simulink model "MAXPID_modelisation_multi_physique_MATLAB_2015a_Ivan_Liebgott"  (R2019b)
settings: Solver=ode15s  StartTime=0.0  StopTime=2.5  RelTol=1e-3  EnableMultiTasking=on
undefined symbols (not defined in the file): sigbuilder_block, X, Y, Z
libraries: sm_lib x140, fl_lib x9, nesl_utility x5, simulink x1, realtime_pacer_lib x1, ee_lib x1
(part 3 of 3)

== system MAXPID_modelisation_multi_physique_MATLAB_2015a_Ivan_Liebgott/Maxpid Simmechanics/bras/AxeArticulation_2_RIGID ==
  ReferenceFrame : sm_lib/Frames and Transforms/Reference Frame
  Solid : sm_lib/Body Elements/File Solid  ExtGeomFileName=AxeArticulation_Défaut_sldprt.STL  UnitType=Custom  ExtGeomFileUnits=mm  StepReaderType=HEX  ExportEntireGeometry=off  InertiaType=Custom  Mass=0.0036367861956118843  MassUnits=kg  CenterOfMass=[0 -0.11402656300615596 2.1307319223985886]  CenterOfMassUnits=mm  MomentsOfInertia=[0.21708338041104236 0.22169225864572503 0.25924252261846747]  MomentsOfInertiaUnits=kg*mm^2  ProductsOfInertia=[-0.0015056290569620979 0 0]  ProductsOfInertiaUnits=kg*mm^2  BasedOnType=Density  Density=1000  DensityUnits=kg/(m^3)  DoExposeReferenceFrame=on  SerializedFrames=<Frames/>  GraphicType=FromGeometry  MarkerShape=Sphere  MarkerSize=10  MarkerSizeUnits=m  GraphicVisPropType=SimpleVisualProperties  GraphicDiffuseColor=[1 1 1]  GraphicSpecularColor=[0.5 0.5 0.5 1.0]  GraphicAmbientColor=[0.15 0.15 0.15 1.0]  GraphicEmissiveColor=[0.0 0.0 0.0 1.0]  GraphicShininess=75  GraphicOpacity=1
  F : PMIOPort  Side=Left
  connections:
  Solid/RConn1 -- ReferenceFrame/RConn1 -- F/RConn1

== system MAXPID_modelisation_multi_physique_MATLAB_2015a_Ivan_Liebgott/Maxpid Simmechanics/bras/AxePoidsVersion95_1_RIGID ==
  ReferenceFrame : sm_lib/Frames and Transforms/Reference Frame
  Solid : sm_lib/Body Elements/File Solid  ExtGeomFileName=AxePoidsVersion95_Défaut_sldprt.STL  UnitType=Custom  ExtGeomFileUnits=mm  StepReaderType=HEX  ExportEntireGeometry=off  InertiaType=Custom  Mass=0.096685500729314755  MassUnits=kg  CenterOfMass=[-4.1541055520205505 9.4534863101010345 -2.6439442480407887e-06]  CenterOfMassUnits=mm  MomentsOfInertia=[93.232729776424421 3.2430818156674595 93.233281036376724]  MomentsOfInertiaUnits=kg*mm^2  ProductsOfInertia=[7.9083095888698852e-05 0.00021129534964956041 -0.00076885839968738841]  ProductsOfInertiaUnits=kg*mm^2  BasedOnType=Density  Density=1000  DensityUnits=kg/(m^3)  DoExposeReferenceFrame=on  SerializedFrames=<Frames/>  GraphicType=FromGeometry  MarkerShape=Sphere  MarkerSize=10  MarkerSizeUnits=m  GraphicVisPropType=SimpleVisualProperties  GraphicDiffuseColor=[1 1 1]  GraphicSpecularColor=[0.5 0.5 0.5 1.0]  GraphicAmbientColor=[0.15 0.15 0.15 1.0]  GraphicEmissiveColor=[0.0 0.0 0.0 1.0]  GraphicShininess=75  GraphicOpacity=1
  F : PMIOPort  Side=Left
  connections:
  Solid/RConn1 -- ReferenceFrame/RConn1 -- F/RConn1

== system MAXPID_modelisation_multi_physique_MATLAB_2015a_Ivan_Liebgott/Maxpid Simmechanics/bras/Bras_1_RIGID ==
  ReferenceFrame : sm_lib/Frames and Transforms/Reference Frame
  Solid : sm_lib/Body Elements/File Solid  ExtGeomFileName=Bras_Défaut_sldprt.STL  UnitType=Custom  ExtGeomFileUnits=mm  StepReaderType=HEX  ExportEntireGeometry=off  InertiaType=Custom  Mass=0.9011079992471549  MassUnits=kg  CenterOfMass=[121.52268202090545 -4.969129514901149 -27.999999999999556]  CenterOfMassUnits=mm  MomentsOfInertia=[5859.4002983757091 495.64724839479584 5534.3999493473466]  MomentsOfInertiaUnits=kg*mm^2  ProductsOfInertia=[0 0 -2.0126056616501971]  ProductsOfInertiaUnits=kg*mm^2  BasedOnType=Density  Density=1000  DensityUnits=kg/(m^3)  DoExposeReferenceFrame=on  SerializedFrames=<Frames/>  GraphicType=FromGeometry  MarkerShape=Sphere  MarkerSize=10  MarkerSizeUnits=m  GraphicVisPropType=SimpleVisualProperties  GraphicDiffuseColor=[0.81960784313725488 0.76078431372549016 0.4392156862745098]  GraphicSpecularColor=[0.5 0.5 0.5 1.0]  GraphicAmbientColor=[0.15 0.15 0.15 1.0]  GraphicEmissiveColor=[0.0 0.0 0.0 1.0]  GraphicShininess=75  GraphicOpacity=1
  F : PMIOPort  Side=Left
  connections:
  Solid/RConn1 -- ReferenceFrame/RConn1 -- F/RConn1

== system MAXPID_modelisation_multi_physique_MATLAB_2015a_Ivan_Liebgott/Maxpid Simmechanics/bras/EcrouSerragePoidsVersion95_1_RIGID ==
  ReferenceFrame : sm_lib/Frames and Transforms/Reference Frame
  Solid : sm_lib/Body Elements/File Solid  ExtGeomFileName=EcrouSerragePoidsVersion95_Défaut_sldprt.STL  UnitType=Custom  ExtGeomFileUnits=mm  StepReaderType=HEX  ExportEntireGeometry=off  InertiaType=Custom  Mass=0.0011915826288096164  MassUnits=kg  CenterOfMass=[3.6591475952271751e-05 -2.9997024398795644 2.6109734489698903e-05]  CenterOfMassUnits=mm  MomentsOfInertia=[0.044097243109792766 0.081206985228529774 0.044103727646083481]  MomentsOfInertiaUnits=kg*mm^2  ProductsOfInertia=[-9.7831064797223504e-09 -4.0511661691424276e-07 8.2961530731377495e-08]  ProductsOfInertiaUnits=kg*mm^2  BasedOnType=Density  Density=1000  DensityUnits=kg/(m^3)  DoExposeReferenceFrame=on  SerializedFrames=<Frames/>  GraphicType=FromGeometry  MarkerShape=Sphere  MarkerSize=10  MarkerSizeUnits=m  GraphicVisPropType=SimpleVisualProperties  GraphicDiffuseColor=[1 1 1]  GraphicSpecularColor=[0.5 0.5 0.5 1.0]  GraphicAmbientColor=[0.15 0.15 0.15 1.0]  GraphicEmissiveColor=[0.0 0.0 0.0 1.0]  GraphicShininess=75  GraphicOpacity=1
  F : PMIOPort  Side=Left
  connections:
  Solid/RConn1 -- ReferenceFrame/RConn1 -- F/RConn1

== system MAXPID_modelisation_multi_physique_MATLAB_2015a_Ivan_Liebgott/Maxpid Simmechanics/bras/EquerreReperage_1_RIGID ==
  ReferenceFrame : sm_lib/Frames and Transforms/Reference Frame
  Solid : sm_lib/Body Elements/File Solid  ExtGeomFileName=EquerreReperage_Défaut_sldprt.STL  UnitType=Custom  ExtGeomFileUnits=mm  StepReaderType=HEX  ExportEntireGeometry=off  InertiaType=Custom  Mass=0.0060891163787629692  MassUnits=kg  CenterOfMass=[19.327887190717206 -10.191107066430515 -0.32701801755483639]  CenterOfMassUnits=mm  MomentsOfInertia=[0.27653523830579496 4.9050369949711774 5.0223555456913935]  MomentsOfInertiaUnits=kg*mm^2  ProductsOfInertia=[0.0086610813542951619 0.27018280182388305 -0.044019297337255049]  ProductsOfInertiaUnits=kg*mm^2  BasedOnType=Density  Density=1000  DensityUnits=kg/(m^3)  DoExposeReferenceFrame=on  SerializedFrames=<Frames/>  GraphicType=FromGeometry  MarkerShape=Sphere  MarkerSize=10  MarkerSizeUnits=m  GraphicVisPropType=SimpleVisualProperties  GraphicDiffuseColor=[1 1 1]  GraphicSpecularColor=[0.5 0.5 0.5 1.0]  GraphicAmbientColor=[0.15 0.15 0.15 1.0]  GraphicEmissiveColor=[0.0 0.0 0.0 1.0]  GraphicShininess=75  GraphicOpacity=1
  F : PMIOPort  Side=Left
  connections:
  Solid/RConn1 -- ReferenceFrame/RConn1 -- F/RConn1

== system MAXPID_modelisation_multi_physique_MATLAB_2015a_Ivan_Liebgott/Maxpid Simmechanics/bras/Poids_1_RIGID ==
  ReferenceFrame : sm_lib/Frames and Transforms/Reference Frame
  Solid : sm_lib/Body Elements/File Solid  ExtGeomFileName=Poids_Défaut_sldprt.STL  UnitType=Custom  ExtGeomFileUnits=mm  StepReaderType=HEX  ExportEntireGeometry=off  InertiaType=Custom  Mass=0.650  MassUnits=kg  CenterOfMass=[-2.0536539050800409 -5.9999999999999618 0]  CenterOfMassUnits=mm  MomentsOfInertia=[161.5932918969379 300.75369148604494 144.75824563880531]  MomentsOfInertiaUnits=kg*mm^2  ProductsOfInertia=[0 0 0]  ProductsOfInertiaUnits=kg*mm^2  BasedOnType=Density  Density=1000  DensityUnits=kg/(m^3)  DoExposeReferenceFrame=on  SerializedFrames=<Frames/>  GraphicType=FromGeometry  MarkerShape=Sphere  MarkerSize=10  MarkerSizeUnits=m  GraphicVisPropType=SimpleVisualProperties  GraphicDiffuseColor=[1 1 1]  GraphicSpecularColor=[0.5 0.5 0.5 1.0]  GraphicAmbientColor=[0.15 0.15 0.15 1.0]  GraphicEmissiveColor=[0.0 0.0 0.0 1.0]  GraphicShininess=75  GraphicOpacity=1
  F : PMIOPort  Side=Left
  connections:
  Solid/RConn1 -- ReferenceFrame/RConn1 -- F/RConn1

== system MAXPID_modelisation_multi_physique_MATLAB_2015a_Ivan_Liebgott/Maxpid Simmechanics/bras/Poids_2_RIGID ==
  ReferenceFrame : sm_lib/Frames and Transforms/Reference Frame
  Solid : sm_lib/Body Elements/File Solid  ExtGeomFileName=Poids_Défaut_sldprt.STL  UnitType=Custom  ExtGeomFileUnits=mm  StepReaderType=HEX  ExportEntireGeometry=off  InertiaType=Custom  Mass=0.650  MassUnits=kg  CenterOfMass=[-2.0536539050800409 -5.9999999999999618 0]  CenterOfMassUnits=mm  MomentsOfInertia=[161.5932918969379 300.75369148604494 144.75824563880531]  MomentsOfInertiaUnits=kg*mm^2  ProductsOfInertia=[0 0 0]  ProductsOfInertiaUnits=kg*mm^2  BasedOnType=Density  Density=1000  DensityUnits=kg/(m^3)  DoExposeReferenceFrame=on  SerializedFrames=<Frames/>  GraphicType=FromGeometry  MarkerShape=Sphere  MarkerSize=10  MarkerSizeUnits=m  GraphicVisPropType=SimpleVisualProperties  GraphicDiffuseColor=[1 1 1]  GraphicSpecularColor=[0.5 0.5 0.5 1.0]  GraphicAmbientColor=[0.15 0.15 0.15 1.0]  GraphicEmissiveColor=[0.0 0.0 0.0 1.0]  GraphicShininess=75  GraphicOpacity=1
  F : PMIOPort  Side=Left
  connections:
  ReferenceFrame/RConn1 -- Solid/RConn1 -- F/RConn1

== system MAXPID_modelisation_multi_physique_MATLAB_2015a_Ivan_Liebgott/Maxpid Simmechanics/bras/Poids_3_RIGID ==
  ReferenceFrame : sm_lib/Frames and Transforms/Reference Frame
  Solid : sm_lib/Body Elements/File Solid  ExtGeomFileName=Poids_Défaut_sldprt.STL  UnitType=Custom  ExtGeomFileUnits=mm  StepReaderType=HEX  ExportEntireGeometry=off  InertiaType=Custom  Mass=0.23324358540409745  MassUnits=kg  CenterOfMass=[-2.0536539050800409 -5.9999999999999618 0]  CenterOfMassUnits=mm  MomentsOfInertia=[161.5932918969379 300.75369148604494 144.75824563880531]  MomentsOfInertiaUnits=kg*mm^2  ProductsOfInertia=[0 0 0]  ProductsOfInertiaUnits=kg*mm^2  BasedOnType=Density  Density=1000  DensityUnits=kg/(m^3)  DoExposeReferenceFrame=on  SerializedFrames=<Frames/>  GraphicType=FromGeometry  MarkerShape=Sphere  MarkerSize=10  MarkerSizeUnits=m  GraphicVisPropType=SimpleVisualProperties  GraphicDiffuseColor=[1 1 1]  GraphicSpecularColor=[0.5 0.5 0.5 1.0]  GraphicAmbientColor=[0.15 0.15 0.15 1.0]  GraphicEmissiveColor=[0.0 0.0 0.0 1.0]  GraphicShininess=75  GraphicOpacity=1
  F : PMIOPort  Side=Left
  connections:
  Solid/RConn1 -- ReferenceFrame/RConn1 -- F/RConn1

== system MAXPID_modelisation_multi_physique_MATLAB_2015a_Ivan_Liebgott/Maxpid Simmechanics/bras/VisChcM4_1_RIGID ==
  ReferenceFrame : sm_lib/Frames and Transforms/Reference Frame
  Solid : sm_lib/Body Elements/File Solid  ExtGeomFileName=VisChcM4_Défaut_sldprt.STL  UnitType=Custom  ExtGeomFileUnits=mm  StepReaderType=HEX  ExportEntireGeometry=off  InertiaType=Custom  Mass=0.0001913087125687861  MassUnits=kg  CenterOfMass=[0.00017482716988745045 3.2099175360591674e-05 -1.3211998133732603]  CenterOfMassUnits=mm  MomentsOfInertia=[0.002318900951955138 0.0023194992151932842 0.00085125281105334291]  MomentsOfInertiaUnits=kg*mm^2  ProductsOfInertia=[-1.9338700142885616e-08 -1.0774030341030306e-07 -2.3956480256821217e-08]  ProductsOfInertiaUnits=kg*mm^2  BasedOnType=Density  Density=1000  DensityUnits=kg/(m^3)  DoExposeReferenceFrame=on  SerializedFrames=<Frames/>  GraphicType=FromGeometry  MarkerShape=Sphere  MarkerSize=10  MarkerSizeUnits=m  GraphicVisPropType=SimpleVisualProperties  GraphicDiffuseColor=[1 1 1]  GraphicSpecularColor=[0.5 0.5 0.5 1.0]  GraphicAmbientColor=[0.15 0.15 0.15 1.0]  GraphicEmissiveColor=[0.0 0.0 0.0 1.0]  GraphicShininess=75  GraphicOpacity=1
  F : PMIOPort  Side=Left
  connections:
  Solid/RConn1 -- ReferenceFrame/RConn1 -- F/RConn1

== system MAXPID_modelisation_multi_physique_MATLAB_2015a_Ivan_Liebgott/Maxpid Simmechanics/bras/VisChcM4_2_RIGID ==
  ReferenceFrame : sm_lib/Frames and Transforms/Reference Frame
  Solid : sm_lib/Body Elements/File Solid  ExtGeomFileName=VisChcM4_Défaut_sldprt.STL  UnitType=Custom  ExtGeomFileUnits=mm  StepReaderType=HEX  ExportEntireGeometry=off  InertiaType=Custom  Mass=0.0001913087125687861  MassUnits=kg  CenterOfMass=[0.00017482716988745045 3.2099175360591674e-05 -1.3211998133732603]  CenterOfMassUnits=mm  MomentsOfInertia=[0.002318900951955138 0.0023194992151932842 0.00085125281105334291]  MomentsOfInertiaUnits=kg*mm^2  ProductsOfInertia=[-1.9338700142885616e-08 -1.0774030341030306e-07 -2.3956480256821217e-08]  ProductsOfInertiaUnits=kg*mm^2  BasedOnType=Density  Density=1000  DensityUnits=kg/(m^3)  DoExposeReferenceFrame=on  SerializedFrames=<Frames/>  GraphicType=FromGeometry  MarkerShape=Sphere  MarkerSize=10  MarkerSizeUnits=m  GraphicVisPropType=SimpleVisualProperties  GraphicDiffuseColor=[1 1 1]  GraphicSpecularColor=[0.5 0.5 0.5 1.0]  GraphicAmbientColor=[0.15 0.15 0.15 1.0]  GraphicEmissiveColor=[0.0 0.0 0.0 1.0]  GraphicShininess=75  GraphicOpacity=1
  F : PMIOPort  Side=Left
  connections:
  Solid/RConn1 -- ReferenceFrame/RConn1 -- F/RConn1

== system MAXPID_modelisation_multi_physique_MATLAB_2015a_Ivan_Liebgott/Maxpid Simmechanics/bras/VisChcM4_3_RIGID ==
  ReferenceFrame : sm_lib/Frames and Transforms/Reference Frame
  Solid : sm_lib/Body Elements/File Solid  ExtGeomFileName=VisChcM4_Défaut_sldprt.STL  UnitType=Custom  ExtGeomFileUnits=mm  StepReaderType=HEX  ExportEntireGeometry=off  InertiaType=Custom  Mass=0.0001913087125687861  MassUnits=kg  CenterOfMass=[0.00017482716988745045 3.2099175360591674e-05 -1.3211998133732603]  CenterOfMassUnits=mm  MomentsOfInertia=[0.002318900951955138 0.0023194992151932842 0.00085125281105334291]  MomentsOfInertiaUnits=kg*mm^2  ProductsOfInertia=[-1.9338700142885616e-08 -1.0774030341030306e-07 -2.3956480256821217e-08]  ProductsOfInertiaUnits=kg*mm^2  BasedOnType=Density  Density=1000  DensityUnits=kg/(m^3)  DoExposeReferenceFrame=on  SerializedFrames=<Frames/>  GraphicType=FromGeometry  MarkerShape=Sphere  MarkerSize=10  MarkerSizeUnits=m  GraphicVisPropType=SimpleVisualProperties  GraphicDiffuseColor=[1 1 1]  GraphicSpecularColor=[0.5 0.5 0.5 1.0]  GraphicAmbientColor=[0.15 0.15 0.15 1.0]  GraphicEmissiveColor=[0.0 0.0 0.0 1.0]  GraphicShininess=75  GraphicOpacity=1
  F : PMIOPort  Side=Left
  connections:
  Solid/RConn1 -- ReferenceFrame/RConn1 -- F/RConn1

== system MAXPID_modelisation_multi_physique_MATLAB_2015a_Ivan_Liebgott/Maxpid Simmechanics/bras/VisChcM4_4_RIGID ==
  ReferenceFrame : sm_lib/Frames and Transforms/Reference Frame
  Solid : sm_lib/Body Elements/File Solid  ExtGeomFileName=VisChcM4_Défaut_sldprt.STL  UnitType=Custom  ExtGeomFileUnits=mm  StepReaderType=HEX  ExportEntireGeometry=off  InertiaType=Custom  Mass=0.0001913087125687861  MassUnits=kg  CenterOfMass=[0.00017482716988745045 3.2099175360591674e-05 -1.3211998133732603]  CenterOfMassUnits=mm  MomentsOfInertia=[0.002318900951955138 0.0023194992151932842 0.00085125281105334291]  MomentsOfInertiaUnits=kg*mm^2  ProductsOfInertia=[-1.9338700142885616e-08 -1.0774030341030306e-07 -2.3956480256821217e-08]  ProductsOfInertiaUnits=kg*mm^2  BasedOnType=Density  Density=1000  DensityUnits=kg/(m^3)  DoExposeReferenceFrame=on  SerializedFrames=<Frames/>  GraphicType=FromGeometry  MarkerShape=Sphere  MarkerSize=10  MarkerSizeUnits=m  GraphicVisPropType=SimpleVisualProperties  GraphicDiffuseColor=[1 1 1]  GraphicSpecularColor=[0.5 0.5 0.5 1.0]  GraphicAmbientColor=[0.15 0.15 0.15 1.0]  GraphicEmissiveColor=[0.0 0.0 0.0 1.0]  GraphicShininess=75  GraphicOpacity=1
  F : PMIOPort  Side=Left
  connections:
  Solid/RConn1 -- ReferenceFrame/RConn1 -- F/RConn1

== system MAXPID_modelisation_multi_physique_MATLAB_2015a_Ivan_Liebgott/Maxpid Simmechanics/bâti/AxeArticulation_1_RIGID ==
  ReferenceFrame : sm_lib/Frames and Transforms/Reference Frame
  Solid : sm_lib/Body Elements/File Solid  ExtGeomFileName=AxeArticulation_Défaut_sldprt.STL  UnitType=Custom  ExtGeomFileUnits=mm  StepReaderType=HEX  ExportEntireGeometry=off  InertiaType=Custom  Mass=0.0036367861956118843  MassUnits=kg  CenterOfMass=[0 -0.11402656300615596 2.1307319223985886]  CenterOfMassUnits=mm  MomentsOfInertia=[0.21708338041104236 0.22169225864572503 0.25924252261846747]  MomentsOfInertiaUnits=kg*mm^2  ProductsOfInertia=[-0.0015056290569620979 0 0]  ProductsOfInertiaUnits=kg*mm^2  BasedOnType=Density  Density=1000  DensityUnits=kg/(m^3)  DoExposeReferenceFrame=on  SerializedFrames=<Frames/>  GraphicType=FromGeometry  MarkerShape=Sphere  MarkerSize=10  MarkerSizeUnits=m  GraphicVisPropType=SimpleVisualProperties  GraphicDiffuseColor=[1 1 1]  GraphicSpecularColor=[0.5 0.5 0.5 1.0]  GraphicAmbientColor=[0.15 0.15 0.15 1.0]  GraphicEmissiveColor=[0.0 0.0 0.0 1.0]  GraphicShininess=75  GraphicOpacity=1
  F : PMIOPort  Side=Left
  connections:
  Solid/RConn1 -- ReferenceFrame/RConn1 -- F/RConn1

== system MAXPID_modelisation_multi_physique_MATLAB_2015a_Ivan_Liebgott/Maxpid Simmechanics/bâti/AxeArticulation_2_RIGID ==
  ReferenceFrame : sm_lib/Frames and Transforms/Reference Frame
  Solid : sm_lib/Body Elements/File Solid  ExtGeomFileName=AxeArticulation_Défaut_sldprt.STL  UnitType=Custom  ExtGeomFileUnits=mm  StepReaderType=HEX  ExportEntireGeometry=off  InertiaType=Custom  Mass=0.0036367861956118843  MassUnits=kg  CenterOfMass=[0 -0.11402656300615596 2.1307319223985886]  CenterOfMassUnits=mm  MomentsOfInertia=[0.21708338041104236 0.22169225864572503 0.25924252261846747]  MomentsOfInertiaUnits=kg*mm^2  ProductsOfInertia=[-0.0015056290569620979 0 0]  ProductsOfInertiaUnits=kg*mm^2  BasedOnType=Density  Density=1000  DensityUnits=kg/(m^3)  DoExposeReferenceFrame=on  SerializedFrames=<Frames/>  GraphicType=FromGeometry  MarkerShape=Sphere  MarkerSize=10  MarkerSizeUnits=m  GraphicVisPropType=SimpleVisualProperties  GraphicDiffuseColor=[1 1 1]  GraphicSpecularColor=[0.5 0.5 0.5 1.0]  GraphicAmbientColor=[0.15 0.15 0.15 1.0]  GraphicEmissiveColor=[0.0 0.0 0.0 1.0]  GraphicShininess=75  GraphicOpacity=1
  F : PMIOPort  Side=Left
  connections:
  Solid/RConn1 -- ReferenceFrame/RConn1 -- F/RConn1

== system MAXPID_modelisation_multi_physique_MATLAB_2015a_Ivan_Liebgott/Maxpid Simmechanics/bâti/AxeBras_1_RIGID ==
  ReferenceFrame : sm_lib/Frames and Transforms/Reference Frame
  Solid : sm_lib/Body Elements/File Solid  ExtGeomFileName=AxeBras_Défaut_sldprt.STL  UnitType=Custom  ExtGeomFileUnits=mm  StepReaderType=HEX  ExportEntireGeometry=off  InertiaType=Custom  Mass=0.065992676097002712  MassUnits=kg  CenterOfMass=[-48.219059130186587 0 0]  CenterOfMassUnits=mm  MomentsOfInertia=[7.4534196241053454 51.91450544053221 51.839580222850827]  MomentsOfInertiaUnits=kg*mm^2  ProductsOfInertia=[0 0 0]  ProductsOfInertiaUnits=kg*mm^2  BasedOnType=Density  Density=1000  DensityUnits=kg/(m^3)  DoExposeReferenceFrame=on  SerializedFrames=<Frames/>  GraphicType=FromGeometry  MarkerShape=Sphere  MarkerSize=10  MarkerSizeUnits=m  GraphicVisPropType=SimpleVisualProperties  GraphicDiffuseColor=[1 1 1]  GraphicSpecularColor=[0.5 0.5 0.5 1.0]  GraphicAmbientColor=[0.15 0.15 0.15 1.0]  GraphicEmissiveColor=[0.0 0.0 0.0 1.0]  GraphicShininess=75  GraphicOpacity=1
  F : PMIOPort  Side=Left
  connections:
  Solid/RConn1 -- ReferenceFrame/RConn1 -- F/RConn1

== system MAXPID_modelisation_multi_physique_MATLAB_2015a_Ivan_Liebgott/Maxpid Simmechanics/bâti/BagueIna30_1_RIGID ==
  ReferenceFrame : sm_lib/Frames and Transforms/Reference Frame
  Solid : sm_lib/Body Elements/File Solid  ExtGeomFileName=BagueIna30_Défaut_sldprt.STL  UnitType=Custom  ExtGeomFileUnits=mm  StepReaderType=HEX  ExportEntireGeometry=off  InertiaType=Custom  Mass=0.0041154863762026296  MassUnits=kg  CenterOfMass=[0 0 5.2290076335877904]  CenterOfMassUnits=mm  MomentsOfInertia=[0.67448569364454569 0.67448569364454569 1.1187054359800583]  MomentsOfInertiaUnits=kg*mm^2  ProductsOfInertia=[0 0 0]  ProductsOfInertiaUnits=kg*mm^2  BasedOnType=Density  Density=1000  DensityUnits=kg/(m^3)  DoExposeReferenceFrame=on  SerializedFrames=<Frames/>  GraphicType=FromGeometry  MarkerShape=Sphere  MarkerSize=10  MarkerSizeUnits=m  GraphicVisPropType=SimpleVisualProperties  GraphicDiffuseColor=[1 1 1]  GraphicSpecularColor=[0.5 0.5 0.5 1.0]  GraphicAmbientColor=[0.15 0.15 0.15 1.0]  GraphicEmissiveColor=[0.0 0.0 0.0 1.0]  GraphicShininess=75  GraphicOpacity=1
  F : PMIOPort  Side=Left
  connections:
  Solid/RConn1 -- ReferenceFrame/RConn1 -- F/RConn1

== system MAXPID_modelisation_multi_physique_MATLAB_2015a_Ivan_Liebgott/Maxpid Simmechanics/bâti/BagueIna30_2_RIGID ==
  ReferenceFrame : sm_lib/Frames and Transforms/Reference Frame
  Solid : sm_lib/Body Elements/File Solid  ExtGeomFileName=BagueIna30_Défaut_sldprt.STL  UnitType=Custom  ExtGeomFileUnits=mm  StepReaderType=HEX  ExportEntireGeometry=off  InertiaType=Custom  Mass=0.0041154863762026296  MassUnits=kg  CenterOfMass=[0 0 5.2290076335877904]  CenterOfMassUnits=mm  MomentsOfInertia=[0.67448569364454569 0.67448569364454569 1.1187054359800583]  MomentsOfInertiaUnits=kg*mm^2  ProductsOfInertia=[0 0 0]  ProductsOfInertiaUnits=kg*mm^2  BasedOnType=Density  Density=1000  DensityUnits=kg/(m^3)  DoExposeReferenceFrame=on  SerializedFrames=<Frames/>  GraphicType=FromGeometry  MarkerShape=Sphere  MarkerSize=10  MarkerSizeUnits=m  GraphicVisPropType=SimpleVisualProperties  GraphicDiffuseColor=[1 1 1]  GraphicSpecularColor=[0.5 0.5 0.5 1.0]  GraphicAmbientColor=[0.15 0.15 0.15 1.0]  GraphicEmissiveColor=[0.0 0.0 0.0 1.0]  GraphicShininess=75  GraphicOpacity=1
  F : PMIOPort  Side=Left
  connections:
  Solid/RConn1 -- ReferenceFrame/RConn1 -- F/RConn1

== system MAXPID_modelisation_multi_physique_MATLAB_2015a_Ivan_Liebgott/Maxpid Simmechanics/bâti/Chaise_2_RIGID ==
  ReferenceFrame : sm_lib/Frames and Transforms/Reference Frame
  Solid : sm_lib/Body Elements/File Solid  ExtGeomFileName=Chaise_Défaut_sldprt.STL  UnitType=Custom  ExtGeomFileUnits=mm  StepReaderType=HEX  ExportEntireGeometry=off  InertiaType=Custom  Mass=0.63330866132065655  MassUnits=kg  CenterOfMass=[-36.098942755399101 -23.213282269439961 3.4449046384098136]  CenterOfMassUnits=mm  MomentsOfInertia=[1238.6670399484537 1348.1802068058498 1548.7516217435766]  MomentsOfInertiaUnits=kg*mm^2  ProductsOfInertia=[-49.85960926730889 -78.757870903878967 251.48102725885036]  ProductsOfInertiaUnits=kg*mm^2  BasedOnType=Density  Density=1000  DensityUnits=kg/(m^3)  DoExposeReferenceFrame=on  SerializedFrames=<Frames/>  GraphicType=FromGeometry  MarkerShape=Sphere  MarkerSize=10  MarkerSizeUnits=m  GraphicVisPropType=SimpleVisualProperties  GraphicDiffuseColor=[1 1 1]  GraphicSpecularColor=[0.5 0.5 0.5 1.0]  GraphicAmbientColor=[0.15 0.15 0.15 1.0]  GraphicEmissiveColor=[0.0 0.0 0.0 1.0]  GraphicShininess=75  GraphicOpacity=1
  F : PMIOPort  Side=Left
  connections:
  Solid/RConn1 -- ReferenceFrame/RConn1 -- F/RConn1

== system MAXPID_modelisation_multi_physique_MATLAB_2015a_Ivan_Liebgott/Maxpid Simmechanics/bâti/VisChcM4_1_RIGID ==
  ReferenceFrame : sm_lib/Frames and Transforms/Reference Frame
  Solid : sm_lib/Body Elements/File Solid  ExtGeomFileName=VisChcM4_Défaut_sldprt.STL  UnitType=Custom  ExtGeomFileUnits=mm  StepReaderType=HEX  ExportEntireGeometry=off  InertiaType=Custom  Mass=0.0001913087125687861  MassUnits=kg  CenterOfMass=[0.00017482716988745045 3.2099175360591674e-05 -1.3211998133732603]  CenterOfMassUnits=mm  MomentsOfInertia=[0.002318900951955138 0.0023194992151932842 0.00085125281105334291]  MomentsOfInertiaUnits=kg*mm^2  ProductsOfInertia=[-1.9338700142885616e-08 -1.0774030341030306e-07 -2.3956480256821217e-08]  ProductsOfInertiaUnits=kg*mm^2  BasedOnType=Density  Density=1000  DensityUnits=kg/(m^3)  DoExposeReferenceFrame=on  SerializedFrames=<Frames/>  GraphicType=FromGeometry  MarkerShape=Sphere  MarkerSize=10  MarkerSizeUnits=m  GraphicVisPropType=SimpleVisualProperties  GraphicDiffuseColor=[1 1 1]  GraphicSpecularColor=[0.5 0.5 0.5 1.0]  GraphicAmbientColor=[0.15 0.15 0.15 1.0]  GraphicEmissiveColor=[0.0 0.0 0.0 1.0]  GraphicShininess=75  GraphicOpacity=1
  F : PMIOPort  Side=Left
  connections:
  Solid/RConn1 -- ReferenceFrame/RConn1 -- F/RConn1

== system MAXPID_modelisation_multi_physique_MATLAB_2015a_Ivan_Liebgott/Maxpid Simmechanics/bâti/VisChcM4_2_RIGID ==
  ReferenceFrame : sm_lib/Frames and Transforms/Reference Frame
  Solid : sm_lib/Body Elements/File Solid  ExtGeomFileName=VisChcM4_Défaut_sldprt.STL  UnitType=Custom  ExtGeomFileUnits=mm  StepReaderType=HEX  ExportEntireGeometry=off  InertiaType=Custom  Mass=0.0001913087125687861  MassUnits=kg  CenterOfMass=[0.00017482716988745045 3.2099175360591674e-05 -1.3211998133732603]  CenterOfMassUnits=mm  MomentsOfInertia=[0.002318900951955138 0.0023194992151932842 0.00085125281105334291]  MomentsOfInertiaUnits=kg*mm^2  ProductsOfInertia=[-1.9338700142885616e-08 -1.0774030341030306e-07 -2.3956480256821217e-08]  ProductsOfInertiaUnits=kg*mm^2  BasedOnType=Density  Density=1000  DensityUnits=kg/(m^3)  DoExposeReferenceFrame=on  SerializedFrames=<Frames/>  GraphicType=FromGeometry  MarkerShape=Sphere  MarkerSize=10  MarkerSizeUnits=m  GraphicVisPropType=SimpleVisualProperties  GraphicDiffuseColor=[1 1 1]  GraphicSpecularColor=[0.5 0.5 0.5 1.0]  GraphicAmbientColor=[0.15 0.15 0.15 1.0]  GraphicEmissiveColor=[0.0 0.0 0.0 1.0]  GraphicShininess=75  GraphicOpacity=1
  F : PMIOPort  Side=Left
  connections:
  Solid/RConn1 -- ReferenceFrame/RConn1 -- F/RConn1

== system MAXPID_modelisation_multi_physique_MATLAB_2015a_Ivan_Liebgott/Maxpid Simmechanics/stator moteur/BagueExtRoulement_1_RIGID ==
  ReferenceFrame : sm_lib/Frames and Transforms/Reference Frame
  Solid : sm_lib/Body Elements/File Solid  ExtGeomFileName=BagueExtRoulement_Défaut_sldprt.STL  UnitType=Custom  ExtGeomFileUnits=mm  StepReaderType=HEX  ExportEntireGeometry=off  InertiaType=Custom  Mass=0.0038510450768364092  MassUnits=kg  CenterOfMass=[7.0000319510488431 -8.0599678600116995e-05 0.00011093594041884269]  CenterOfMassUnits=mm  MomentsOfInertia=[0.69336925634395152 0.41405877280178383 0.41405877282416026]  MomentsOfInertiaUnits=kg*mm^2  ProductsOfInertia=[0 2.6350463662162988e-06 -1.9144732483385565e-06]  ProductsOfInertiaUnits=kg*mm^2  BasedOnType=Density  Density=1000  DensityUnits=kg/(m^3)  DoExposeReferenceFrame=on  SerializedFrames=<Frames/>  GraphicType=FromGeometry  MarkerShape=Sphere  MarkerSize=10  MarkerSizeUnits=m  GraphicVisPropType=SimpleVisualProperties  GraphicDiffuseColor=[1 1 1]  GraphicSpecularColor=[0.5 0.5 0.5 1.0]  GraphicAmbientColor=[0.15 0.15 0.15 1.0]  GraphicEmissiveColor=[0.0 0.0 0.0 1.0]  GraphicShininess=75  GraphicOpacity=1
  F : PMIOPort  Side=Left
  connections:
  Solid/RConn1 -- ReferenceFrame/RConn1 -- F/RConn1

== system MAXPID_modelisation_multi_physique_MATLAB_2015a_Ivan_Liebgott/Maxpid Simmechanics/stator moteur/BrideMoteur_1_RIGID ==
  ReferenceFrame : sm_lib/Frames and Transforms/Reference Frame
  Solid : sm_lib/Body Elements/File Solid  ExtGeomFileName=BrideMoteur_Défaut_sldprt.STL  UnitType=Custom  ExtGeomFileUnits=mm  StepReaderType=HEX  ExportEntireGeometry=off  InertiaType=Custom  Mass=0.0072375749754014819  MassUnits=kg  CenterOfMass=[-0.75805962995788589 0 0]  CenterOfMassUnits=mm  MomentsOfInertia=[2.0200946460825637 1.0328876994622069 1.0221175830303963]  MomentsOfInertiaUnits=kg*mm^2  ProductsOfInertia=[0.016573505017822766 0 0]  ProductsOfInertiaUnits=kg*mm^2  BasedOnType=Density  Density=1000  DensityUnits=kg/(m^3)  DoExposeReferenceFrame=on  SerializedFrames=<Frames/>  GraphicType=FromGeometry  MarkerShape=Sphere  MarkerSize=10  MarkerSizeUnits=m  GraphicVisPropType=SimpleVisualProperties  GraphicDiffuseColor=[1 1 1]  GraphicSpecularColor=[0.5 0.5 0.5 1.0]  GraphicAmbientColor=[0.15 0.15 0.15 1.0]  GraphicEmissiveColor=[0.0 0.0 0.0 1.0]  GraphicShininess=75  GraphicOpacity=1
  F : PMIOPort  Side=Left
  connections:
  Solid/RConn1 -- ReferenceFrame/RConn1 -- F/RConn1

== system MAXPID_modelisation_multi_physique_MATLAB_2015a_Ivan_Liebgott/Maxpid Simmechanics/stator moteur/EcrouSupportVisBille_1_RIGID ==
  ReferenceFrame : sm_lib/Frames and Transforms/Reference Frame
  Solid : sm_lib/Body Elements/File Solid  ExtGeomFileName=EcrouSupportVisBille_Défaut_sldprt.STL  UnitType=Custom  ExtGeomFileUnits=mm  StepReaderType=HEX  ExportEntireGeometry=off  InertiaType=Custom  Mass=0.010448937165840137  MassUnits=kg  CenterOfMass=[-2.333132892363301 0 0]  CenterOfMassUnits=mm  MomentsOfInertia=[4.4530900908984696 2.4304273571172446 2.430427357117245]  MomentsOfInertiaUnits=kg*mm^2  ProductsOfInertia=[0 0 0]  ProductsOfInertiaUnits=kg*mm^2  BasedOnType=Density  Density=1000  DensityUnits=kg/(m^3)  DoExposeReferenceFrame=on  SerializedFrames=<Frames/>  GraphicType=FromGeometry  MarkerShape=Sphere  MarkerSize=10  MarkerSizeUnits=m  GraphicVisPropType=SimpleVisualProperties  GraphicDiffuseColor=[1 1 1]  GraphicSpecularColor=[0.5 0.5 0.5 1.0]  GraphicAmbientColor=[0.15 0.15 0.15 1.0]  GraphicEmissiveColor=[0.0 0.0 0.0 1.0]  GraphicShininess=75  GraphicOpacity=1
  F : PMIOPort  Side=Left
  connections:
  Solid/RConn1 -- ReferenceFrame/RConn1 -- F/RConn1

== system MAXPID_modelisation_multi_physique_MATLAB_2015a_Ivan_Liebgott/Maxpid Simmechanics/stator moteur/StatorMoteur_1_RIGID ==
  ReferenceFrame : sm_lib/Frames and Transforms/Reference Frame
  Solid : sm_lib/Body Elements/File Solid  ExtGeomFileName=StatorMoteur_Défaut_sldprt.STL  UnitType=Custom  ExtGeomFileUnits=mm  StepReaderType=HEX  ExportEntireGeometry=off  InertiaType=Custom  Mass=0.046775958417462925  MassUnits=kg  CenterOfMass=[-40.071570092516247 0 0]  CenterOfMassUnits=mm  MomentsOfInertia=[8.8878119375048996 34.005816311117478 34.005816311117478]  MomentsOfInertiaUnits=kg*mm^2  ProductsOfInertia=[0 0 0]  ProductsOfInertiaUnits=kg*mm^2  BasedOnType=Density  Density=1000  DensityUnits=kg/(m^3)  DoExposeReferenceFrame=on  SerializedFrames=<Frames/>  GraphicType=FromGeometry  MarkerShape=Sphere  MarkerSize=10  MarkerSizeUnits=m  GraphicVisPropType=SimpleVisualProperties  GraphicDiffuseColor=[0.54117647058823526 0.61960784313725492 0.63529411764705879]  GraphicSpecularColor=[0.5 0.5 0.5 1.0]  GraphicAmbientColor=[0.15 0.15 0.15 1.0]  GraphicEmissiveColor=[0.0 0.0 0.0 1.0]  GraphicShininess=75  GraphicOpacity=1
  F : PMIOPort  Side=Left
  connections:
  Solid/RConn1 -- ReferenceFrame/RConn1 -- F/RConn1

== system MAXPID_modelisation_multi_physique_MATLAB_2015a_Ivan_Liebgott/Maxpid Simmechanics/stator moteur/SupprotVisBille_1_RIGID ==
  ReferenceFrame : sm_lib/Frames and Transforms/Reference Frame
  Solid : sm_lib/Body Elements/File Solid  ExtGeomFileName=SupprotVisBille_Défaut_sldprt.STL  UnitType=Custom  ExtGeomFileUnits=mm  StepReaderType=HEX  ExportEntireGeometry=off  InertiaType=Custom  Mass=0.065858964727791208  MassUnits=kg  CenterOfMass=[-21.219204181038744 9.0724322775499953e-05 6.9647184094116462e-05]  CenterOfMassUnits=mm  MomentsOfInertia=[25.288316413205944 28.456398698867311 29.096770221577124]  MomentsOfInertiaUnits=kg*mm^2  ProductsOfInertia=[-0.98558179877514163 -1.1505462754503571e-05 -1.0726056129042532e-05]  ProductsOfInertiaUnits=kg*mm^2  BasedOnType=Density  Density=1000  DensityUnits=kg/(m^3)  DoExposeReferenceFrame=on  SerializedFrames=<Frames/>  GraphicType=FromGeometry  MarkerShape=Sphere  MarkerSize=10  MarkerSizeUnits=m  GraphicVisPropType=SimpleVisualProperties  GraphicDiffuseColor=[1 1 1]  GraphicSpecularColor=[0.5 0.5 0.5 1.0]  GraphicAmbientColor=[0.15 0.15 0.15 1.0]  GraphicEmissiveColor=[0.0 0.0 0.0 1.0]  GraphicShininess=75  GraphicOpacity=1
  F : PMIOPort  Side=Left
  connections:
  Solid/RConn1 -- ReferenceFrame/RConn1 -- F/RConn1
